simulink model "SIMQGC"  (R2017a)
settings: Solver=VariableStepAuto  StartTime=0.0  StopTime=1000  RelTol=1e-3
model workspace: external: MAT-File (data not in the file)
values from neighbouring files (symbols this model uses):
  aDe =     [MY3.mat]
  aDyn =     [MY3.mat]
  aLat =     [MY3.mat]
  aLon =     [MY3.mat]
  H = HGround + geo.Zgear + GearData.R - MCdata.mass*9.8/4/GearData.Sp    [my3_acdata.m]
  HGround = 500    [my3_acdata.m]
  phi_max = 20    [my3_acdata.m]
  phi_min = -20    [my3_acdata.m]
  psi_max = 30    [my3_acdata.m]
  psi_min = -30    [my3_acdata.m]
  theta_max = 20    [my3_acdata.m]
  theta_min = -20    [my3_acdata.m]
  Xmax = 0.01    [my3_acdata.m]
  Xmin = 0    [my3_acdata.m]
  Ymax = 0.01    [my3_acdata.m]
  Ymin = 0    [my3_acdata.m]
  Zmax = 0.01    [my3_acdata.m]
  Zmin = 0    [my3_acdata.m]
undefined symbols (not defined in the file or in its folder): Earth, geo, ini, magnitude, Motor, Newton, Prop, Raphson, Standard_Devices, UDP_Protocol, WGS84
undefined symbols (not defined in the file): GearData, LProp, RProp
libraries: simulink_extras x12, dspnetwork x8, aerolibobsolete x6, sharedutil x6, simulink x4, aerolibfltsims x3, aerolibasang x2, aerolibatmos2 x1, aerolibbdyn x1, aerolibtransform2 x1, aerolibanimutils x1, sldrtlib x1
(part 3 of 3)

== system SIMQGC/AircraftModel_MY3/Fixwing_Airframe/GroundForces/RF_Gear/detect ground contact ==
  note: height of gear lowest point
  ze : Inport
  DCM : Inport  Port=2
  Xgb : Inport  Port=3
  Hrw : Inport  Port=4
  Gain2 : Gain  Gain=-1
  Rotate pos to body axes : Product  Multiplication=Matrix(*)  SaturateOnIntegerOverflow=on  InputSameDT=on  OutDataTypeStr=Inherit: Same as first input
  Sum2 : Sum  Inputs=|++
  Sum4 : Sum  Inputs=++|
  Transpose : Math  Operator=transpose  SaturateOnIntegerOverflow=on
  Zg : Selector  InputPortWidth=3  IndexOptions=Index vector (dialog)  Indices=3  OutputSizes=1
  detect_WOW : RelationalOperator  Operator=<=  OutDataTypeStr=boolean  RndMeth=Nearest
  radius of wheel : Constant  Value=Rw  VectorParams1D=off
  WOW : Outport
  wires:
  radius of wheel/1 -> Sum2/2
  Transpose/1 -> Rotate pos to body axes/1
  Zg/1 -> Sum4/2
  Gain2/1 -> detect_WOW/1
  Sum2/1 -> Gain2/1
  Sum4/1 -> Sum2/1
  Rotate pos to body axes/1 -> Zg/1
  DCM/1 -> Transpose/1
  Xgb/1 -> Rotate pos to body axes/2
  Hrw/1 -> detect_WOW/2
  ze/1 -> Sum4/1
  detect_WOW/1 -> WOW/1

== system SIMQGC/AircraftModel_MY3/Fixwing_Airframe/PlantBus/nb & gb /cal gb ==
  DCM : Inport
  g : Inport  Port=2
  Constant2 : Constant  Value=0
  Mux : Mux  Inputs=3
  To Body Axes : Product  Multiplication=Matrix(*)  SaturateOnIntegerOverflow=on  InputSameDT=on  OutDataTypeStr=Inherit: Same as first input
  gb : Outport
  wires:
  Mux/1 -> To Body Axes/2
  Constant2/1 -> Mux/1, Mux/2
  DCM/1 -> To Body Axes/1
  To Body Axes/1 -> gb/1
  g/1 -> Mux/3

== system SIMQGC/AircraftModel_MY3/Fixwing_Airframe/Aerodynamics/Aerodynamic Coefficients/Basic Coefficients/alat ==
  beta : Inport
  alpha : Inport  Port=2
  Mux : Mux  Inputs=6
  alat_CD : Lookup_n-D  BreakpointsForDimension1=aLat.beta  BreakpointsForDimension2=aLat.alpha  Table=aLat.dCD  InternalRulePriority=Speed  RndMeth=Simplest  InputSameDT=on
  alat_CL : Lookup_n-D  BreakpointsForDimension1=aLat.beta  BreakpointsForDimension2=aLat.alpha  Table=aLat.dCL  InternalRulePriority=Speed  RndMeth=Simplest  InputSameDT=on
  alat_CY : Lookup_n-D  BreakpointsForDimension1=aLat.beta  BreakpointsForDimension2=aLat.alpha  Table=aLat.dCY  InternalRulePriority=Speed  RndMeth=Simplest  InputSameDT=on
  alat_Cl : Lookup_n-D  BreakpointsForDimension1=aLat.beta  BreakpointsForDimension2=aLat.alpha  Table=aLat.dCl  InternalRulePriority=Speed  RndMeth=Simplest  InputSameDT=on
  alat_Cm : Lookup_n-D  BreakpointsForDimension1=aLat.beta  BreakpointsForDimension2=aLat.alpha  Table=aLat.dCm  InternalRulePriority=Speed  RndMeth=Simplest  InputSameDT=on
  alat_Cn : Lookup_n-D  BreakpointsForDimension1=aLat.beta  BreakpointsForDimension2=aLat.alpha  Table=aLat.dCn  InternalRulePriority=Speed  RndMeth=Simplest  InputSameDT=on
  alat : Outport
  wires:
  beta/1 -> alat_Cn/1, alat_Cm/1, alat_Cl/1, alat_CY/1, alat_CD/1, alat_CL/1
  alpha/1 -> alat_Cn/2, alat_Cm/2, alat_Cl/2, alat_CY/2, alat_CD/2, alat_CL/2
  alat_Cm/1 -> Mux/5
  alat_CD/1 -> Mux/2
  alat_CL/1 -> Mux/1
  Mux/1 -> alat/1
  alat_CY/1 -> Mux/3
  alat_Cl/1 -> Mux/4
  alat_Cn/1 -> Mux/6

== system SIMQGC/AircraftModel_MY3/Fixwing_Airframe/Aerodynamics/Aerodynamic Coefficients/Basic Coefficients/alon ==
  alpha : Inport
  Mach : Inport  Port=2
  Constant : Constant  Value=0
  Constant1 : Constant  Value=0
  Constant2 : Constant  Value=0
  Mux : Mux  Inputs=6
  alon_CD : Lookup_n-D  BreakpointsForDimension1=aLon.alpha  BreakpointsForDimension2=aLon.mach  Table=aLon.CD  InternalRulePriority=Speed  RndMeth=Simplest  InputSameDT=on
  alon_CL : Lookup_n-D  BreakpointsForDimension1=aLon.alpha  BreakpointsForDimension2=aLon.mach  Table=aLon.CL  InternalRulePriority=Speed  RndMeth=Simplest  InputSameDT=on
  alon_Cm : Lookup_n-D  BreakpointsForDimension1=aLon.alpha  BreakpointsForDimension2=aLon.mach  Table=aLon.Cm  InternalRulePriority=Speed  RndMeth=Simplest  InputSameDT=on
  alon : Outport
  wires:
  Mux/1 -> alon/1
  alon_CL/1 -> Mux/1
  alon_CD/1 -> Mux/2
  alon_Cm/1 -> Mux/5
  Mach/1 -> alon_CL/2, alon_Cm/2, alon_CD/2
  alpha/1 -> alon_CL/1, alon_Cm/1, alon_CD/1
  Constant/1 -> Mux/3
  Constant1/1 -> Mux/4
  Constant2/1 -> Mux/6

== system SIMQGC/AircraftModel_MY3/Fixwing_Airframe/Aerodynamics/Aerodynamic Coefficients/Body Rate Damping/adyn ==
  alpha : Inport
  adyn_p : Subsystem
  adyn_q : Subsystem
  adyn_r : Subsystem
  pout : Outport
  qout : Outport  Port=2
  rout : Outport  Port=3
  wires:
  alpha/1 -> adyn_r/1(alpha), adyn_q/1(alpha), adyn_p/1(alpha)
  adyn_p/1(p) -> pout/1
  adyn_q/1(q) -> qout/1
  adyn_r/1(r) -> rout/1

== system SIMQGC/AircraftModel_MY3/Fixwing_Airframe/Aerodynamics/Aerodynamic Coefficients/actuator/ade ==
  alpha : Inport
  de : Inport  Port=2
  CD : Lookup_n-D  BreakpointsForDimension1=aDe.de  BreakpointsForDimension2=aDe.alpha  Table=aDe.dCD  InternalRulePriority=Speed  RndMeth=Simplest  InputSameDT=on
  CL : Lookup_n-D  BreakpointsForDimension1=aDe.de  BreakpointsForDimension2=aDe.alpha  Table=aDe.dCL  InternalRulePriority=Speed  RndMeth=Simplest  InputSameDT=on
  Cm : Lookup_n-D  BreakpointsForDimension1=aDe.de  BreakpointsForDimension2=aDe.alpha  Table=aDe.dCm  InternalRulePriority=Speed  RndMeth=Simplest  InputSameDT=on
  Mux2 : Mux  Inputs=6
  cld_height : Constant  Value=0
  Coeff : Outport
  wires:
  Mux2/1 -> Coeff/1
  de/1 -> Cm/1, CD/1, CL/1
  alpha/1 -> Cm/2, CD/2, CL/2
  CL/1 -> Mux2/1
  CD/1 -> Mux2/2
  cld_height/1 -> Mux2/4, Mux2/6, Mux2/3
  Cm/1 -> Mux2/5

== system SIMQGC/AircraftModel_MY3/Fixwing_Airframe/Aerodynamics/DerivedConditions1/Incidence, Sideslip, & Airspeed/Subsystem ==
  V : Inport
  Demux1 : Demux  Outputs=3
  Terminator : Terminator
  w : Outport
  U : Outport  Port=2
  wires:
  Demux1/3 -> w/1
  Demux1/2 -> Terminator/1
  V/1 -> Demux1/1
  Demux1/1 -> U/1

== system SIMQGC/AircraftModel_MY3/Fixwing_Airframe/Aerodynamics/DerivedConditions1/Incidence, Sideslip, & Airspeed/Subsystem1 ==
  V : Inport
  Demux1 : Demux  Outputs=3
  Terminator : Terminator
  Terminator1 : Terminator
  v : Outport
  wires:
  Demux1/1 -> Terminator/1
  Demux1/3 -> Terminator1/1
  V/1 -> Demux1/1
  Demux1/2 -> v/1

== system SIMQGC/AircraftModel_MY3/Fixwing_Airframe/Aerodynamics/DerivedConditions1/Incidence, Sideslip, & Airspeed/dot ==
  Vb : Inport
  Demux1 : Demux  Outputs=3
  Product : Product  RndMeth=Zero
  Product1 : Product  RndMeth=Zero
  Product2 : Product  RndMeth=Zero
  Sum : Sum  Inputs=+++
  dot : Outport
  wires:
  Product2/1 -> Sum/3
  Demux1/3 -> Product2/2, Product2/1
  Product/1 -> Sum/1
  Product1/1 -> Sum/2
  Sum/1 -> dot/1
  Vb/1 -> Demux1/1
  Demux1/1 -> Product/2, Product/1
  Demux1/2 -> Product1/1, Product1/2

== system SIMQGC/AircraftModel_MY3/Fixwing_Airframe/Aerodynamics/DerivedConditions1/gamma chi & speed/norm ==
  x : Inport
  y : Inport  Port=2
  z : Inport  Port=3
  Product1 : Product  RndMeth=Zero
  Product2 : Product  RndMeth=Zero
  Product3 : Product  RndMeth=Zero
  Sum : Sum  Inputs=+++
  speed : Math  Operator=sqrt  SaturateOnIntegerOverflow=on
  n : Outport
  wires:
  Product3/1 -> Sum/3
  Product1/1 -> Sum/1
  Product2/1 -> Sum/2
  Sum/1 -> speed/1
  speed/1 -> n/1
  x/1 -> Product1/1, Product1/2
  y/1 -> Product2/1, Product2/2
  z/1 -> Product3/1, Product3/2

== system SIMQGC/AircraftModel_MY3/Fixwing_Airframe/GroundForces/LF_Gear/GenerateGroundFM1/Calc Gear Force and Pos ==
  Xgb : Inport
  zrw : Inport  Port=2
  zcg : Inport  Port=3
  DCM : Inport  Port=4
  WgL : Inport  Port=5
  DampingRate_N/m/sec1 : Gain  Gain=Cs
  Product : Product  Multiplication=Matrix(*)
  Selector : Selector  InputPortWidth=3  IndexOptions=Index vector (dialog)  Indices=[3]  OutputSizes=1
  Selector1 : Selector  InputPortWidth=3  IndexOptions=Index vector (dialog)  Indices=[3]  OutputSizes=1
  SpringRate_N/m1 : Gain  Gain=Ks
  Sum : Sum  Inputs=+--
  Sum4 : Sum  Inputs=|-+
  Sum5 : Sum
  Transpose1 : Math  Operator=transpose  SaturateOnIntegerOverflow=on
  radius of  wheel1 : Constant  Value=Rw  VectorParams1D=off
  reaction1 : Gain  Gain=-1
  Fz1 : Outport
  S_strut1 : Outport  Port=2  InitialOutput=0
  zgb1 : Outport  Port=3  InitialOutput=0
  wires:
  DCM/1 -> Transpose1/1
  Xgb/1 -> Selector1/1, Product/2
  Transpose1/1 -> Product/1
  Product/1 -> Selector/1
  Selector/1 -> Sum/3
  zcg/1 -> Sum/2
  zrw/1 -> Sum/1
  Sum/1 -> Sum4/1
  radius of  wheel1/1 -> Sum4/2
  SpringRate_N/m1/1 -> Sum5/1
  WgL/1 -> DampingRate_N/m/sec1/1
  DampingRate_N/m/sec1/1 -> Sum5/2
  Sum5/1 -> reaction1/1  "Fstrut"
  reaction1/1 -> Fz1/1
  Selector1/1 -> zgb1/1
  Sum4/1 -> S_strut1/1, SpringRate_N/m1/1

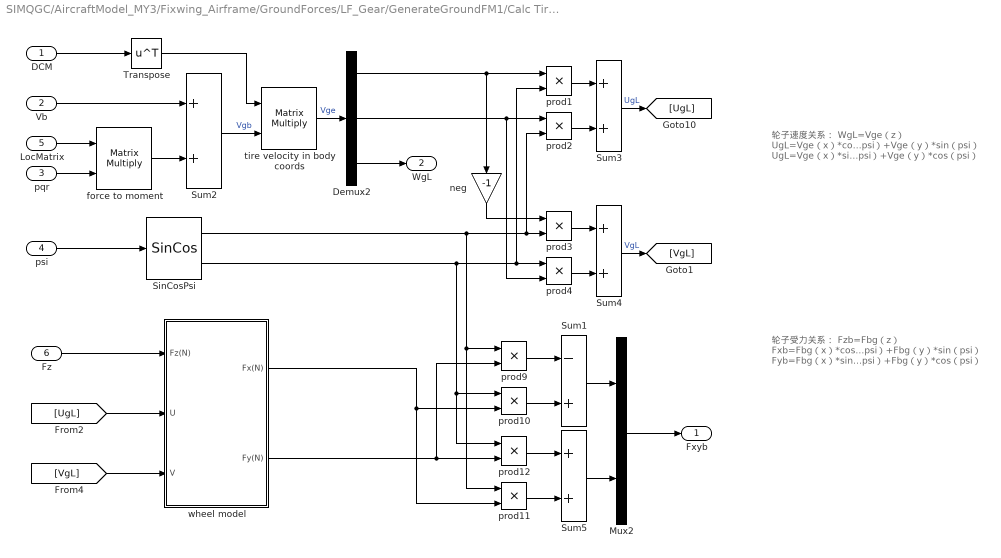
== system SIMQGC/AircraftModel_MY3/Fixwing_Airframe/GroundForces/LF_Gear/GenerateGroundFM1/Calc Tire Force ==
  note: 轮子速度关系：
      | WgL=Vge（z）
      | UgL=Vge（x）*cos（psi）+Vge（y）*sin（psi）
      | UgL=Vge（x）*sin（psi）+Vge（y）*cos（psi）
  note: 轮子受力关系：
      | Fzb=Fbg（z）
      | Fxb=Fbg（x）*cos（psi）+Fbg（y）*sin（psi）
      | Fyb=Fbg（x）*sin（psi）+Fbg（y）*cos（psi）
  DCM : Inport
  Vb : Inport  Port=2
  pqr : Inport  Port=3
  psi : Inport  Port=4
  LocMatrix : Inport  Port=5
  Fz : Inport  Port=6
  Demux2 : Demux  Outputs=3
  Mux2 : Mux  Inputs=2
  SinCosPsi : aerolibobsolete/SinCos
      settings: SourceProductName=Aerospace Blockset  SourceProductBaseCode=AE
  Sum1 : Sum  Inputs=-+
  Sum2 : Sum  Inputs=2
  Sum3 : Sum  Inputs=2
  Sum4 : Sum  Inputs=2
  Sum5 : Sum
  Transpose : Math  Operator=transpose  SaturateOnIntegerOverflow=on
  force to moment : Product  Multiplication=Matrix(*)  SaturateOnIntegerOverflow=on  InputSameDT=on  OutDataTypeStr=Inherit: Same as first input
  neg : Gain  Gain=-1
  prod{1..4,9..12} (8 alike) : Product  RndMeth=Zero
  tire velocity in body coords : Product  Multiplication=Matrix(*)  SaturateOnIntegerOverflow=on  InputSameDT=on  OutDataTypeStr=Inherit: Same as first input
  wheel model : Subsystem
  Fxyb : Outport  InitialOutput=0
  WgL : Outport  Port=2  InitialOutput=0
  wires:
  psi/1 -> SinCosPsi/1
  Sum4/1 -> [VgL]  "VgL"
  [VgL] -> wheel model/3(V)
  [UgL] -> wheel model/2(U)
  Mux2/1 -> Fxyb/1
  Sum5/1 -> Mux2/2
  Sum1/1 -> Mux2/1
  prod11/1 -> Sum5/2
  prod12/1 -> Sum5/1
  prod10/1 -> Sum1/2
  prod9/1 -> Sum1/1
  force to moment/1 -> Sum2/2
  Sum2/1 -> tire velocity in body coords/2  "Vgb"
  tire velocity in body coords/1 -> Demux2/1  "Vge"
  Demux2/1 -> neg/1, prod1/1
  Demux2/2 -> prod2/1, prod4/2
  prod1/1 -> Sum3/1
  prod2/1 -> Sum3/2
  prod3/1 -> Sum4/1
  prod4/1 -> Sum4/2
  Sum3/1 -> [UgL]  "UgL"
  neg/1 -> prod3/1
  SinCosPsi/1 -> prod11/1, prod9/1, prod2/2, prod3/2
  SinCosPsi/2 -> prod12/1, prod10/1, prod1/2, prod4/1
  Vb/1 -> Sum2/1
  LocMatrix/1 -> force to moment/1
  pqr/1 -> force to moment/2
  DCM/1 -> Transpose/1
  Transpose/1 -> tire velocity in body coords/1
  wheel model/1(Fx(N)) -> prod11/2, prod10/2
  wheel model/2(Fy(N)) -> prod9/2, prod12/2
  Fz/1 -> wheel model/1(Fz(N))
  Demux2/3 -> WgL/1

== system SIMQGC/AircraftModel_MY3/Fixwing_Airframe/GroundForces/LF_Gear/GenerateGroundFM1/LocMatrix ==
  xgb : Inport
  ygb : Inport  Port=2
  zgb : Inport  Port=3
  Create 3x3 Matrix : sharedutil/Create 3x3 Matrix
  Sum : Sum  Inputs=++|
  inv1 : Gain  Gain=-1
  inv2 : Gain  Gain=-1
  inv4 : Gain  Gain=-1
  zero1 : Constant  Value=0  SampleTime=0
  zero2 : Constant  Value=0  SampleTime=0
  zero3 : Constant  Value=0  SampleTime=0
  zero4 : Constant  Value=Rw  SampleTime=0
  A : Outport
  wires:
  xgb/1 -> Create 3x3 Matrix/6, inv2/1
  ygb/1 -> inv1/1, Create 3x3 Matrix/7
  Create 3x3 Matrix/1 -> A/1
  zero1/1 -> Create 3x3 Matrix/1
  zero2/1 -> Create 3x3 Matrix/5
  zero3/1 -> Create 3x3 Matrix/9
  inv1/1 -> Create 3x3 Matrix/3
  inv4/1 -> Create 3x3 Matrix/4
  inv2/1 -> Create 3x3 Matrix/8
  zgb/1 -> Sum/2
  zero4/1 -> Sum/1
  Sum/1 -> inv4/1, Create 3x3 Matrix/2

== system SIMQGC/AircraftModel_MY3/Fixwing_Airframe/GroundForces/LM_Gear/GenerateGroundFM1/Calc Gear Force and Pos ==
  Xgb : Inport
  zrg : Inport  Port=2
  zcg : Inport  Port=3
  DCM : Inport  Port=4
  WgL : Inport  Port=5
  DampingRate_N/m/sec1 : Gain  Gain=Cs
  Product : Product  Multiplication=Matrix(*)
  Selector : Selector  InputPortWidth=3  IndexOptions=Index vector (dialog)  Indices=[3]  OutputSizes=1
  Selector1 : Selector  InputPortWidth=3  IndexOptions=Index vector (dialog)  Indices=[3]  OutputSizes=1
  SpringRate_N/m1 : Gain  Gain=Ks
  Sum : Sum  Inputs=+--
  Sum4 : Sum  Inputs=|-+
  Sum5 : Sum
  Transpose1 : Math  Operator=transpose  SaturateOnIntegerOverflow=on
  radius of  wheel1 : Constant  Value=Rw  VectorParams1D=off
  reaction1 : Gain  Gain=-1
  Fz1 : Outport
  S_strut1 : Outport  Port=2  InitialOutput=0
  zgb1 : Outport  Port=3  InitialOutput=0
  wires:
  DCM/1 -> Transpose1/1
  Xgb/1 -> Selector1/1, Product/2
  Transpose1/1 -> Product/1
  Product/1 -> Selector/1
  Selector/1 -> Sum/3
  zcg/1 -> Sum/2
  zrg/1 -> Sum/1
  Sum/1 -> Sum4/1
  radius of  wheel1/1 -> Sum4/2
  SpringRate_N/m1/1 -> Sum5/1
  WgL/1 -> DampingRate_N/m/sec1/1
  DampingRate_N/m/sec1/1 -> Sum5/2
  Sum5/1 -> reaction1/1  "Fstrut"
  reaction1/1 -> Fz1/1
  Selector1/1 -> zgb1/1
  Sum4/1 -> S_strut1/1, SpringRate_N/m1/1

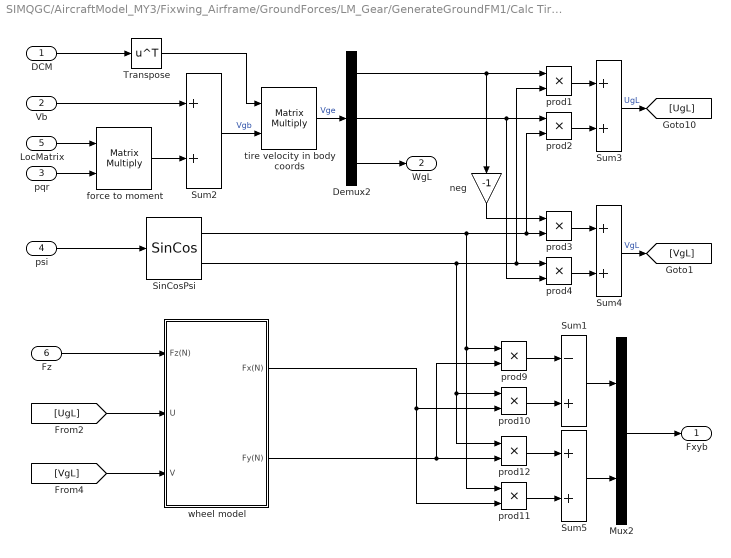
== system SIMQGC/AircraftModel_MY3/Fixwing_Airframe/GroundForces/LM_Gear/GenerateGroundFM1/Calc Tire Force ==
  DCM : Inport
  Vb : Inport  Port=2
  pqr : Inport  Port=3
  psi : Inport  Port=4
  LocMatrix : Inport  Port=5
  Fz : Inport  Port=6
  Demux2 : Demux  Outputs=3
  Mux2 : Mux  Inputs=2
  SinCosPsi : aerolibobsolete/SinCos
      settings: SourceProductName=Aerospace Blockset  SourceProductBaseCode=AE
  Sum1 : Sum  Inputs=-+
  Sum2 : Sum  Inputs=2
  Sum3 : Sum  Inputs=2
  Sum4 : Sum  Inputs=2
  Sum5 : Sum
  Transpose : Math  Operator=transpose  SaturateOnIntegerOverflow=on
  force to moment : Product  Multiplication=Matrix(*)  SaturateOnIntegerOverflow=on  InputSameDT=on  OutDataTypeStr=Inherit: Same as first input
  neg : Gain  Gain=-1
  prod{1..4,9..12} (8 alike) : Product  RndMeth=Zero
  tire velocity in body coords : Product  Multiplication=Matrix(*)  SaturateOnIntegerOverflow=on  InputSameDT=on  OutDataTypeStr=Inherit: Same as first input
  wheel model : Subsystem
  Fxyb : Outport  InitialOutput=0
  WgL : Outport  Port=2  InitialOutput=0
  wires:
  psi/1 -> SinCosPsi/1
  Sum4/1 -> [VgL]  "VgL"
  [VgL] -> wheel model/3(V)
  [UgL] -> wheel model/2(U)
  Mux2/1 -> Fxyb/1
  Sum5/1 -> Mux2/2
  Sum1/1 -> Mux2/1
  prod11/1 -> Sum5/2
  prod12/1 -> Sum5/1
  prod10/1 -> Sum1/2
  prod9/1 -> Sum1/1
  force to moment/1 -> Sum2/2
  Sum2/1 -> tire velocity in body coords/2  "Vgb"
  tire velocity in body coords/1 -> Demux2/1  "Vge"
  Demux2/1 -> neg/1, prod1/1
  Demux2/2 -> prod2/1, prod4/2
  prod1/1 -> Sum3/1
  prod2/1 -> Sum3/2
  prod3/1 -> Sum4/1
  prod4/1 -> Sum4/2
  Sum3/1 -> [UgL]  "UgL"
  neg/1 -> prod3/1
  SinCosPsi/1 -> prod11/1, prod9/1, prod2/2, prod3/2
  SinCosPsi/2 -> prod12/1, prod10/1, prod1/2, prod4/1
  Vb/1 -> Sum2/1
  LocMatrix/1 -> force to moment/1
  pqr/1 -> force to moment/2
  DCM/1 -> Transpose/1
  Transpose/1 -> tire velocity in body coords/1
  wheel model/1(Fx(N)) -> prod11/2, prod10/2
  wheel model/2(Fy(N)) -> prod9/2, prod12/2
  Fz/1 -> wheel model/1(Fz(N))
  Demux2/3 -> WgL/1

== system SIMQGC/AircraftModel_MY3/Fixwing_Airframe/GroundForces/LM_Gear/GenerateGroundFM1/LocMatrix ==
  xgb : Inport
  ygb : Inport  Port=2
  zgb : Inport  Port=3
  Create 3x3 Matrix : sharedutil/Create 3x3 Matrix
  Sum : Sum  Inputs=++|
  inv1 : Gain  Gain=-1
  inv2 : Gain  Gain=-1
  inv4 : Gain  Gain=-1
  zero1 : Constant  Value=0  SampleTime=0
  zero2 : Constant  Value=0  SampleTime=0
  zero3 : Constant  Value=0  SampleTime=0
  zero4 : Constant  Value=Rw  SampleTime=0
  A : Outport
  wires:
  xgb/1 -> Create 3x3 Matrix/6, inv2/1
  ygb/1 -> inv1/1, Create 3x3 Matrix/7
  Create 3x3 Matrix/1 -> A/1
  zero1/1 -> Create 3x3 Matrix/1
  zero2/1 -> Create 3x3 Matrix/5
  zero3/1 -> Create 3x3 Matrix/9
  inv1/1 -> Create 3x3 Matrix/3
  inv4/1 -> Create 3x3 Matrix/4
  inv2/1 -> Create 3x3 Matrix/8
  zgb/1 -> Sum/2
  zero4/1 -> Sum/1
  Sum/1 -> inv4/1, Create 3x3 Matrix/2

== system SIMQGC/AircraftModel_MY3/Fixwing_Airframe/GroundForces/LN_Gear/GenerateGroundFM1/Calc Gear Force and Pos ==
  Xgb : Inport
  zrg : Inport  Port=2
  zcg : Inport  Port=3
  DCM : Inport  Port=4
  WgL : Inport  Port=5
  DampingRate_N/m/sec1 : Gain  Gain=Cs
  Product : Product  Multiplication=Matrix(*)
  Selector : Selector  InputPortWidth=3  IndexOptions=Index vector (dialog)  Indices=[3]  OutputSizes=1
  Selector1 : Selector  InputPortWidth=3  IndexOptions=Index vector (dialog)  Indices=[3]  OutputSizes=1
  SpringRate_N/m1 : Gain  Gain=Ks
  Sum : Sum  Inputs=+--
  Sum4 : Sum  Inputs=|-+
  Sum5 : Sum
  Transpose1 : Math  Operator=transpose  SaturateOnIntegerOverflow=on
  radius of  wheel1 : Constant  Value=Rw  VectorParams1D=off
  reaction1 : Gain  Gain=-1
  Fz1 : Outport
  S_strut1 : Outport  Port=2  InitialOutput=0
  zgb1 : Outport  Port=3  InitialOutput=0
  wires:
  DCM/1 -> Transpose1/1
  Xgb/1 -> Selector1/1, Product/2
  Transpose1/1 -> Product/1
  Product/1 -> Selector/1
  Selector/1 -> Sum/3
  zcg/1 -> Sum/2
  zrg/1 -> Sum/1
  Sum/1 -> Sum4/1
  radius of  wheel1/1 -> Sum4/2
  SpringRate_N/m1/1 -> Sum5/1
  WgL/1 -> DampingRate_N/m/sec1/1
  DampingRate_N/m/sec1/1 -> Sum5/2
  Sum5/1 -> reaction1/1  "Fstrut"
  reaction1/1 -> Fz1/1
  Selector1/1 -> zgb1/1
  Sum4/1 -> S_strut1/1, SpringRate_N/m1/1

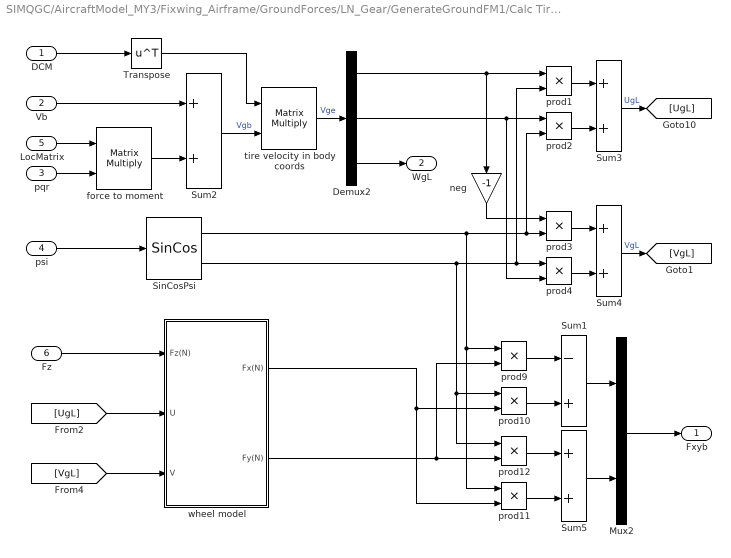
== system SIMQGC/AircraftModel_MY3/Fixwing_Airframe/GroundForces/LN_Gear/GenerateGroundFM1/Calc Tire Force ==
  DCM : Inport
  Vb : Inport  Port=2
  pqr : Inport  Port=3
  psi : Inport  Port=4
  LocMatrix : Inport  Port=5
  Fz : Inport  Port=6
  Demux2 : Demux  Outputs=3
  Mux2 : Mux  Inputs=2
  SinCosPsi : aerolibobsolete/SinCos
      settings: SourceProductName=Aerospace Blockset  SourceProductBaseCode=AE
  Sum1 : Sum  Inputs=-+
  Sum2 : Sum  Inputs=2
  Sum3 : Sum  Inputs=2
  Sum4 : Sum  Inputs=2
  Sum5 : Sum
  Transpose : Math  Operator=transpose  SaturateOnIntegerOverflow=on
  force to moment : Product  Multiplication=Matrix(*)  SaturateOnIntegerOverflow=on  InputSameDT=on  OutDataTypeStr=Inherit: Same as first input
  neg : Gain  Gain=-1
  prod{1..4,9..12} (8 alike) : Product  RndMeth=Zero
  tire velocity in body coords : Product  Multiplication=Matrix(*)  SaturateOnIntegerOverflow=on  InputSameDT=on  OutDataTypeStr=Inherit: Same as first input
  wheel model : Subsystem
  Fxyb : Outport  InitialOutput=0
  WgL : Outport  Port=2  InitialOutput=0
  wires:
  psi/1 -> SinCosPsi/1
  Sum4/1 -> [VgL]  "VgL"
  [VgL] -> wheel model/3(V)
  [UgL] -> wheel model/2(U)
  Mux2/1 -> Fxyb/1
  Sum5/1 -> Mux2/2
  Sum1/1 -> Mux2/1
  prod11/1 -> Sum5/2
  prod12/1 -> Sum5/1
  prod10/1 -> Sum1/2
  prod9/1 -> Sum1/1
  force to moment/1 -> Sum2/2
  Sum2/1 -> tire velocity in body coords/2  "Vgb"
  tire velocity in body coords/1 -> Demux2/1  "Vge"
  Demux2/1 -> neg/1, prod1/1
  Demux2/2 -> prod2/1, prod4/2
  prod1/1 -> Sum3/1
  prod2/1 -> Sum3/2
  prod3/1 -> Sum4/1
  prod4/1 -> Sum4/2
  Sum3/1 -> [UgL]  "UgL"
  neg/1 -> prod3/1
  SinCosPsi/1 -> prod11/1, prod9/1, prod2/2, prod3/2
  SinCosPsi/2 -> prod12/1, prod10/1, prod1/2, prod4/1
  Vb/1 -> Sum2/1
  LocMatrix/1 -> force to moment/1
  pqr/1 -> force to moment/2
  DCM/1 -> Transpose/1
  Transpose/1 -> tire velocity in body coords/1
  wheel model/1(Fx(N)) -> prod11/2, prod10/2
  wheel model/2(Fy(N)) -> prod9/2, prod12/2
  Fz/1 -> wheel model/1(Fz(N))
  Demux2/3 -> WgL/1

== system SIMQGC/AircraftModel_MY3/Fixwing_Airframe/GroundForces/LN_Gear/GenerateGroundFM1/LocMatrix ==
  xgb : Inport
  ygb : Inport  Port=2
  zgb : Inport  Port=3
  Create 3x3 Matrix : sharedutil/Create 3x3 Matrix
  Sum : Sum  Inputs=++|
  inv1 : Gain  Gain=-1
  inv2 : Gain  Gain=-1
  inv4 : Gain  Gain=-1
  zero1 : Constant  Value=0  SampleTime=0
  zero2 : Constant  Value=0  SampleTime=0
  zero3 : Constant  Value=0  SampleTime=0
  zero4 : Constant  Value=Rw  SampleTime=0
  A : Outport
  wires:
  xgb/1 -> Create 3x3 Matrix/6, inv2/1
  ygb/1 -> inv1/1, Create 3x3 Matrix/7
  Create 3x3 Matrix/1 -> A/1
  zero1/1 -> Create 3x3 Matrix/1
  zero2/1 -> Create 3x3 Matrix/5
  zero3/1 -> Create 3x3 Matrix/9
  inv1/1 -> Create 3x3 Matrix/3
  inv4/1 -> Create 3x3 Matrix/4
  inv2/1 -> Create 3x3 Matrix/8
  zgb/1 -> Sum/2
  zero4/1 -> Sum/1
  Sum/1 -> inv4/1, Create 3x3 Matrix/2

== system SIMQGC/AircraftModel_MY3/Fixwing_Airframe/GroundForces/RF_Gear/GenerateGroundFM1/Calc Gear Force and Pos ==
  Xgb : Inport
  zrg : Inport  Port=2
  zcg : Inport  Port=3
  DCM : Inport  Port=4
  WgL : Inport  Port=5
  DampingRate_N/m/sec1 : Gain  Gain=Cs
  Product : Product  Multiplication=Matrix(*)
  Selector : Selector  InputPortWidth=3  IndexOptions=Index vector (dialog)  Indices=[3]  OutputSizes=1
  Selector1 : Selector  InputPortWidth=3  IndexOptions=Index vector (dialog)  Indices=[3]  OutputSizes=1
  SpringRate_N/m1 : Gain  Gain=Ks
  Sum : Sum  Inputs=+--
  Sum4 : Sum  Inputs=|-+
  Sum5 : Sum
  Transpose1 : Math  Operator=transpose  SaturateOnIntegerOverflow=on
  radius of  wheel1 : Constant  Value=Rw  VectorParams1D=off
  reaction1 : Gain  Gain=-1
  Fz1 : Outport
  S_strut1 : Outport  Port=2  InitialOutput=0
  zgb1 : Outport  Port=3  InitialOutput=0
  wires:
  DCM/1 -> Transpose1/1
  Xgb/1 -> Selector1/1, Product/2
  Transpose1/1 -> Product/1
  Product/1 -> Selector/1
  Selector/1 -> Sum/3
  zcg/1 -> Sum/2
  zrg/1 -> Sum/1
  Sum/1 -> Sum4/1
  radius of  wheel1/1 -> Sum4/2
  SpringRate_N/m1/1 -> Sum5/1
  WgL/1 -> DampingRate_N/m/sec1/1
  DampingRate_N/m/sec1/1 -> Sum5/2
  Sum5/1 -> reaction1/1  "Fstrut"
  reaction1/1 -> Fz1/1
  Selector1/1 -> zgb1/1
  Sum4/1 -> S_strut1/1, SpringRate_N/m1/1

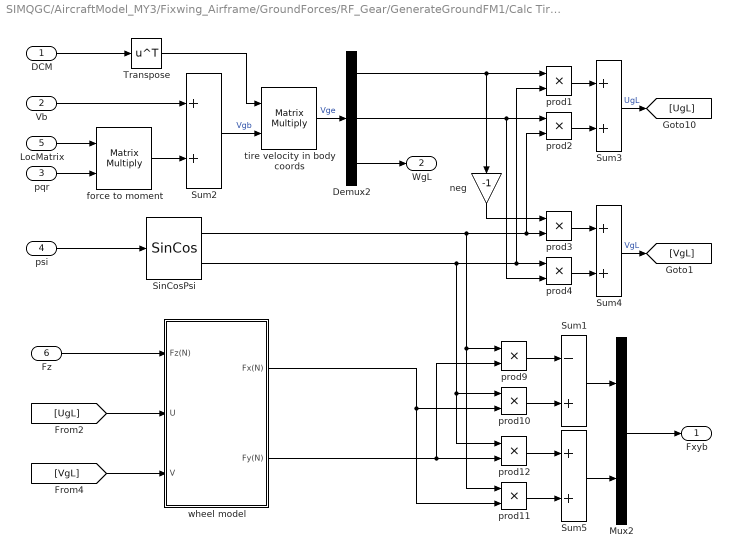
== system SIMQGC/AircraftModel_MY3/Fixwing_Airframe/GroundForces/RF_Gear/GenerateGroundFM1/Calc Tire Force ==
  DCM : Inport
  Vb : Inport  Port=2
  pqr : Inport  Port=3
  psi : Inport  Port=4
  LocMatrix : Inport  Port=5
  Fz : Inport  Port=6
  Demux2 : Demux  Outputs=3
  Mux2 : Mux  Inputs=2
  SinCosPsi : aerolibobsolete/SinCos
      settings: SourceProductName=Aerospace Blockset  SourceProductBaseCode=AE
  Sum1 : Sum  Inputs=-+
  Sum2 : Sum  Inputs=2
  Sum3 : Sum  Inputs=2
  Sum4 : Sum  Inputs=2
  Sum5 : Sum
  Transpose : Math  Operator=transpose  SaturateOnIntegerOverflow=on
  force to moment : Product  Multiplication=Matrix(*)  SaturateOnIntegerOverflow=on  InputSameDT=on  OutDataTypeStr=Inherit: Same as first input
  neg : Gain  Gain=-1
  prod{1..4,9..12} (8 alike) : Product  RndMeth=Zero
  tire velocity in body coords : Product  Multiplication=Matrix(*)  SaturateOnIntegerOverflow=on  InputSameDT=on  OutDataTypeStr=Inherit: Same as first input
  wheel model : Subsystem
  Fxyb : Outport  InitialOutput=0
  WgL : Outport  Port=2  InitialOutput=0
  wires:
  psi/1 -> SinCosPsi/1
  Sum4/1 -> [VgL]  "VgL"
  [VgL] -> wheel model/3(V)
  [UgL] -> wheel model/2(U)
  Mux2/1 -> Fxyb/1
  Sum5/1 -> Mux2/2
  Sum1/1 -> Mux2/1
  prod11/1 -> Sum5/2
  prod12/1 -> Sum5/1
  prod10/1 -> Sum1/2
  prod9/1 -> Sum1/1
  force to moment/1 -> Sum2/2
  Sum2/1 -> tire velocity in body coords/2  "Vgb"
  tire velocity in body coords/1 -> Demux2/1  "Vge"
  Demux2/1 -> neg/1, prod1/1
  Demux2/2 -> prod2/1, prod4/2
  prod1/1 -> Sum3/1
  prod2/1 -> Sum3/2
  prod3/1 -> Sum4/1
  prod4/1 -> Sum4/2
  Sum3/1 -> [UgL]  "UgL"
  neg/1 -> prod3/1
  SinCosPsi/1 -> prod11/1, prod9/1, prod2/2, prod3/2
  SinCosPsi/2 -> prod12/1, prod10/1, prod1/2, prod4/1
  Vb/1 -> Sum2/1
  LocMatrix/1 -> force to moment/1
  pqr/1 -> force to moment/2
  DCM/1 -> Transpose/1
  Transpose/1 -> tire velocity in body coords/1
  wheel model/1(Fx(N)) -> prod11/2, prod10/2
  wheel model/2(Fy(N)) -> prod9/2, prod12/2
  Fz/1 -> wheel model/1(Fz(N))
  Demux2/3 -> WgL/1

== system SIMQGC/AircraftModel_MY3/Fixwing_Airframe/GroundForces/RF_Gear/GenerateGroundFM1/LocMatrix ==
  xgb : Inport
  ygb : Inport  Port=2
  zgb : Inport  Port=3
  Create 3x3 Matrix : sharedutil/Create 3x3 Matrix
  Sum : Sum  Inputs=++|
  inv1 : Gain  Gain=-1
  inv2 : Gain  Gain=-1
  inv4 : Gain  Gain=-1
  zero1 : Constant  Value=0  SampleTime=0
  zero2 : Constant  Value=0  SampleTime=0
  zero3 : Constant  Value=0  SampleTime=0
  zero4 : Constant  Value=Rw  SampleTime=0
  A : Outport
  wires:
  xgb/1 -> Create 3x3 Matrix/6, inv2/1
  ygb/1 -> inv1/1, Create 3x3 Matrix/7
  Create 3x3 Matrix/1 -> A/1
  zero1/1 -> Create 3x3 Matrix/1
  zero2/1 -> Create 3x3 Matrix/5
  zero3/1 -> Create 3x3 Matrix/9
  inv1/1 -> Create 3x3 Matrix/3
  inv4/1 -> Create 3x3 Matrix/4
  inv2/1 -> Create 3x3 Matrix/8
  zgb/1 -> Sum/2
  zero4/1 -> Sum/1
  Sum/1 -> inv4/1, Create 3x3 Matrix/2

== system SIMQGC/AircraftModel_MY3/Fixwing_Airframe/Aerodynamics/Aerodynamic Coefficients/Body Rate Damping/adyn/adyn_p ==
  alpha : Inport
  Constant : Constant  Value=0
  Mux : Mux  Inputs=6
  Yp : Lookup_n-D  NumberOfTableDimensions=1  BreakpointsForDimension1=aDyn.alpha  Table=aDyn.CYp  InternalRulePriority=Speed  RndMeth=Simplest  InputSameDT=on
  lp : Lookup_n-D  NumberOfTableDimensions=1  BreakpointsForDimension1=aDyn.alpha  Table=aDyn.Clp  InternalRulePriority=Speed  RndMeth=Simplest  InputSameDT=on
  np : Lookup_n-D  NumberOfTableDimensions=1  BreakpointsForDimension1=aDyn.alpha  Table=aDyn.Cnp  InternalRulePriority=Speed  RndMeth=Simplest  InputSameDT=on
  p : Outport
  wires:
  lp/1 -> Mux/4
  Yp/1 -> Mux/3
  np/1 -> Mux/6
  alpha/1 -> np/1, lp/1, Yp/1
  Constant/1 -> Mux/1, Mux/2, Mux/5
  Mux/1 -> p/1

== system SIMQGC/AircraftModel_MY3/Fixwing_Airframe/Aerodynamics/Aerodynamic Coefficients/Body Rate Damping/adyn/adyn_q ==
  alpha : Inport
  Constant : Constant  Value=0
  Dq : Lookup_n-D  NumberOfTableDimensions=1  BreakpointsForDimension1=aDyn.alpha  Table=aDyn.CDq  InternalRulePriority=Speed  RndMeth=Simplest  InputSameDT=on
  Lq : Lookup_n-D  NumberOfTableDimensions=1  BreakpointsForDimension1=aDyn.alpha  Table=aDyn.CLq  InternalRulePriority=Speed  RndMeth=Simplest  InputSameDT=on
  Mq : Lookup_n-D  NumberOfTableDimensions=1  BreakpointsForDimension1=aDyn.alpha  Table=aDyn.Cmq  InternalRulePriority=Speed  RndMeth=Simplest  InputSameDT=on
  Mux : Mux  Inputs=6
  q : Outport
  wires:
  Mux/1 -> q/1
  alpha/1 -> Mq/1, Dq/1, Lq/1
  Lq/1 -> Mux/1
  Dq/1 -> Mux/2
  Mq/1 -> Mux/5
  Constant/1 -> Mux/6, Mux/4, Mux/3

== system SIMQGC/AircraftModel_MY3/Fixwing_Airframe/Aerodynamics/Aerodynamic Coefficients/Body Rate Damping/adyn/adyn_r ==
  alpha : Inport
  Constant : Constant  Value=0
  Mux : Mux  Inputs=6
  Yr : Lookup_n-D  NumberOfTableDimensions=1  BreakpointsForDimension1=aDyn.alpha  Table=aDyn.CYr  InternalRulePriority=Speed  RndMeth=Simplest  InputSameDT=on
  lr : Lookup_n-D  NumberOfTableDimensions=1  BreakpointsForDimension1=aDyn.alpha  Table=aDyn.Clr  InternalRulePriority=Speed  RndMeth=Simplest  InputSameDT=on
  nr : Lookup_n-D  NumberOfTableDimensions=1  BreakpointsForDimension1=aDyn.alpha  Table=aDyn.Cnr  InternalRulePriority=Speed  RndMeth=Simplest  InputSameDT=on
  r : Outport
  wires:
  Mux/1 -> r/1
  Constant/1 -> Mux/5, Mux/2, Mux/1
  alpha/1 -> Yr/1, nr/1, lr/1
  nr/1 -> Mux/6
  Yr/1 -> Mux/3
  lr/1 -> Mux/4

== system SIMQGC/AircraftModel_MY3/Fixwing_Airframe/GroundForces/LF_Gear/GenerateGroundFM1/Calc Tire Force/wheel model ==
  note: simple wheel model
      | no wheel model and brake device model
      | not consider slip ratio caused forces
  Fz(N) : Inport
  U : Inport  Port=2
  V : Inport  Port=3
  Abs : Abs  ZeroCross=off
  Abs1 : Abs
  Gain : Gain  Gain=-1
  Gain1 : Gain  Gain=-1
  Gain2 : Gain  Gain=-1
  Product1 : Product  SaturateOnIntegerOverflow=on  InputSameDT=on  OutDataTypeStr=Inherit: Same as first input
  Product2 : Product  SaturateOnIntegerOverflow=on  InputSameDT=on  OutDataTypeStr=Inherit: Same as first input
  Product3 : Product  SaturateOnIntegerOverflow=on  InputSameDT=on  OutDataTypeStr=Inherit: Same as first input
  Saturation : Saturate  UpperLimit=10  LowerLimit=-10
  Sign : Signum  ZeroCross=off
  Switch : Switch  Threshold=0.01  ZeroCross=off
  cal side slipe angle : Subsystem
  lateral force: A*beta*(1-B*beta^2) : Fcn  Expr=A*u[1]*(1-B*u[1]*u[1])
  roll friction conefficient : Constant  Value=muroll
  Fx(N) : Outport
  Fy(N) : Outport  Port=2
  wires:
  Product2/1 -> Fy(N)/1
  Switch/1 -> Fx(N)/1
  Gain1/1 -> Product2/2
  lateral force: A*beta*(1-B*beta^2)/1 -> Gain1/1
  Saturation/1 -> lateral force: A*beta*(1-B*beta^2)/1
  V/1 -> cal side slipe angle/2(v)
  Product1/1 -> Switch/1
  Abs1/1 -> Switch/2
  Gain2/1 -> Switch/3
  Gain/1 -> Product1/2
  Abs/1 -> Product2/1, Product3/2
  Sign/1 -> Gain/1
  Product3/1 -> Product1/1
  U/1 -> cal side slipe angle/1(u), Abs1/1, Gain2/1, Sign/1
  roll friction conefficient/1 -> Product3/1
  Fz(N)/1 -> Abs/1
  cal side slipe angle/1(betae) -> Saturation/1

== system SIMQGC/AircraftModel_MY3/Fixwing_Airframe/GroundForces/LM_Gear/GenerateGroundFM1/Calc Tire Force/wheel model ==
  note: simple wheel model
      | no wheel model and brake device model
      | not consider slip ratio caused forces
  Fz(N) : Inport
  U : Inport  Port=2
  V : Inport  Port=3
  Abs : Abs  ZeroCross=off
  Abs1 : Abs
  Gain : Gain  Gain=-1
  Gain1 : Gain  Gain=-1
  Gain2 : Gain  Gain=-1
  Product1 : Product  SaturateOnIntegerOverflow=on  InputSameDT=on  OutDataTypeStr=Inherit: Same as first input
  Product2 : Product  SaturateOnIntegerOverflow=on  InputSameDT=on  OutDataTypeStr=Inherit: Same as first input
  Product3 : Product  SaturateOnIntegerOverflow=on  InputSameDT=on  OutDataTypeStr=Inherit: Same as first input
  Saturation : Saturate  UpperLimit=10  LowerLimit=-10
  Sign : Signum  ZeroCross=off
  Switch : Switch  Threshold=0.01  ZeroCross=off
  cal side slipe angle : Subsystem
  lateral force: A*beta*(1-B*beta^2) : Fcn  Expr=A*u[1]*(1-B*u[1]*u[1])
  roll friction conefficient : Constant  Value=muroll
  Fx(N) : Outport
  Fy(N) : Outport  Port=2
  wires:
  Product2/1 -> Fy(N)/1
  Switch/1 -> Fx(N)/1
  Gain1/1 -> Product2/2
  lateral force: A*beta*(1-B*beta^2)/1 -> Gain1/1
  Saturation/1 -> lateral force: A*beta*(1-B*beta^2)/1
  V/1 -> cal side slipe angle/2(v)
  Product1/1 -> Switch/1
  Abs1/1 -> Switch/2
  Gain2/1 -> Switch/3
  Gain/1 -> Product1/2
  Abs/1 -> Product2/1, Product3/2
  Sign/1 -> Gain/1
  Product3/1 -> Product1/1
  U/1 -> cal side slipe angle/1(u), Abs1/1, Gain2/1, Sign/1
  roll friction conefficient/1 -> Product3/1
  Fz(N)/1 -> Abs/1
  cal side slipe angle/1(betae) -> Saturation/1

== system SIMQGC/AircraftModel_MY3/Fixwing_Airframe/GroundForces/LN_Gear/GenerateGroundFM1/Calc Tire Force/wheel model ==
  note: simple wheel model
      | no wheel model and brake device model
      | not consider slip ratio caused forces
  Fz(N) : Inport
  U : Inport  Port=2
  V : Inport  Port=3
  Abs : Abs  ZeroCross=off
  Abs1 : Abs
  Gain : Gain  Gain=-1
  Gain1 : Gain  Gain=-1
  Gain2 : Gain  Gain=-1
  Product1 : Product  SaturateOnIntegerOverflow=on  InputSameDT=on  OutDataTypeStr=Inherit: Same as first input
  Product2 : Product  SaturateOnIntegerOverflow=on  InputSameDT=on  OutDataTypeStr=Inherit: Same as first input
  Product3 : Product  SaturateOnIntegerOverflow=on  InputSameDT=on  OutDataTypeStr=Inherit: Same as first input
  Saturation : Saturate  UpperLimit=10  LowerLimit=-10
  Sign : Signum  ZeroCross=off
  Switch : Switch  Threshold=0.01  ZeroCross=off
  cal side slipe angle : Subsystem
  lateral force: A*beta*(1-B*beta^2) : Fcn  Expr=A*u[1]*(1-B*u[1]*u[1])
  roll friction conefficient : Constant  Value=muroll
  Fx(N) : Outport
  Fy(N) : Outport  Port=2
  wires:
  Product2/1 -> Fy(N)/1
  Switch/1 -> Fx(N)/1
  Gain1/1 -> Product2/2
  lateral force: A*beta*(1-B*beta^2)/1 -> Gain1/1
  Saturation/1 -> lateral force: A*beta*(1-B*beta^2)/1
  V/1 -> cal side slipe angle/2(v)
  Product1/1 -> Switch/1
  Abs1/1 -> Switch/2
  Gain2/1 -> Switch/3
  Gain/1 -> Product1/2
  Abs/1 -> Product2/1, Product3/2
  Sign/1 -> Gain/1
  Product3/1 -> Product1/1
  U/1 -> cal side slipe angle/1(u), Abs1/1, Gain2/1, Sign/1
  roll friction conefficient/1 -> Product3/1
  Fz(N)/1 -> Abs/1
  cal side slipe angle/1(betae) -> Saturation/1

== system SIMQGC/AircraftModel_MY3/Fixwing_Airframe/GroundForces/RF_Gear/GenerateGroundFM1/Calc Tire Force/wheel model ==
  note: simple wheel model
      | no wheel model and brake device model
      | not consider slip ratio caused forces
  Fz(N) : Inport
  U : Inport  Port=2
  V : Inport  Port=3
  Abs : Abs  ZeroCross=off
  Abs1 : Abs
  Gain : Gain  Gain=-1
  Gain1 : Gain  Gain=-1
  Gain2 : Gain  Gain=-1
  Product1 : Product  SaturateOnIntegerOverflow=on  InputSameDT=on  OutDataTypeStr=Inherit: Same as first input
  Product2 : Product  SaturateOnIntegerOverflow=on  InputSameDT=on  OutDataTypeStr=Inherit: Same as first input
  Product3 : Product  SaturateOnIntegerOverflow=on  InputSameDT=on  OutDataTypeStr=Inherit: Same as first input
  Saturation : Saturate  UpperLimit=10  LowerLimit=-10
  Sign : Signum  ZeroCross=off
  Switch : Switch  Threshold=0.01  ZeroCross=off
  cal side slipe angle : Subsystem
  lateral force: A*beta*(1-B*beta^2) : Fcn  Expr=A*u[1]*(1-B*u[1]*u[1])
  roll friction conefficient : Constant  Value=muroll
  Fx(N) : Outport
  Fy(N) : Outport  Port=2
  wires:
  Product2/1 -> Fy(N)/1
  Switch/1 -> Fx(N)/1
  Gain1/1 -> Product2/2
  lateral force: A*beta*(1-B*beta^2)/1 -> Gain1/1
  Saturation/1 -> lateral force: A*beta*(1-B*beta^2)/1
  V/1 -> cal side slipe angle/2(v)
  Product1/1 -> Switch/1
  Abs1/1 -> Switch/2
  Gain2/1 -> Switch/3
  Gain/1 -> Product1/2
  Abs/1 -> Product2/1, Product3/2
  Sign/1 -> Gain/1
  Product3/1 -> Product1/1
  U/1 -> cal side slipe angle/1(u), Abs1/1, Gain2/1, Sign/1
  roll friction conefficient/1 -> Product3/1
  Fz(N)/1 -> Abs/1
  cal side slipe angle/1(betae) -> Saturation/1

== system SIMQGC/AircraftModel_MY3/Fixwing_Airframe/GroundForces/LF_Gear/GenerateGroundFM1/Calc Tire Force/wheel model/cal side slipe angle ==
  note: u>0.01
  u : Inport
  v : Inport  Port=2
  Saturation : Saturate  UpperLimit=inf  LowerLimit=1
  Trigonometric Function : Trigonometry  Operator=atan2
  betae : Outport
  wires:
  u/1 -> Saturation/1
  Saturation/1 -> Trigonometric Function/2
  Trigonometric Function/1 -> betae/1
  v/1 -> Trigonometric Function/1

== system SIMQGC/AircraftModel_MY3/Fixwing_Airframe/GroundForces/LM_Gear/GenerateGroundFM1/Calc Tire Force/wheel model/cal side slipe angle ==
  note: u>0.01
  u : Inport
  v : Inport  Port=2
  Saturation : Saturate  UpperLimit=inf  LowerLimit=1
  Trigonometric Function : Trigonometry  Operator=atan2
  betae : Outport
  wires:
  u/1 -> Saturation/1
  Saturation/1 -> Trigonometric Function/2
  Trigonometric Function/1 -> betae/1
  v/1 -> Trigonometric Function/1

== system SIMQGC/AircraftModel_MY3/Fixwing_Airframe/GroundForces/LN_Gear/GenerateGroundFM1/Calc Tire Force/wheel model/cal side slipe angle ==
  note: u>0.01
  u : Inport
  v : Inport  Port=2
  Saturation : Saturate  UpperLimit=inf  LowerLimit=1
  Trigonometric Function : Trigonometry  Operator=atan2
  betae : Outport
  wires:
  u/1 -> Saturation/1
  Saturation/1 -> Trigonometric Function/2
  Trigonometric Function/1 -> betae/1
  v/1 -> Trigonometric Function/1

== system SIMQGC/AircraftModel_MY3/Fixwing_Airframe/GroundForces/RF_Gear/GenerateGroundFM1/Calc Tire Force/wheel model/cal side slipe angle ==
  note: u>0.01
  u : Inport
  v : Inport  Port=2
  Saturation : Saturate  UpperLimit=inf  LowerLimit=1
  Trigonometric Function : Trigonometry  Operator=atan2
  betae : Outport
  wires:
  u/1 -> Saturation/1
  Saturation/1 -> Trigonometric Function/2
  Trigonometric Function/1 -> betae/1
  v/1 -> Trigonometric Function/1

== matlab function SIMQGC/UDPSendToQGC/UDP_send 3 /Byte Pack ==
  data: head input; OUT output; index input; data input
function OUT = data_transfer_uint8(head,index,data)
OUT = uint8(zeros(41,1));
OUT(1 : 5) = uint8(head);
OUT(6) = uint8(index);
OUT(10:41) = typecast(single(data),'uint8');
end

== matlab function SIMQGC/UDPSendToQGC/UDP_send 4/Byte Pack ==
  data: head input; OUT output; index input; data input
function OUT = data_transfer_uint8(head,index,data)
OUT = uint8(zeros(41,1));
OUT(1 : 5) = uint8(head);
OUT(6) = uint8(index);
OUT(10:41) = typecast(single(data),'uint8');
end

== matlab function SIMQGC/UDPSendToQGC/UDP_send 6/Byte Pack ==
  data: head input; OUT output; index input; data input
function OUT = data_transfer_uint8(head,index,data)
OUT = uint8(zeros(41,1));
OUT(1 : 5) = uint8(head);
OUT(6) = uint8(index);
OUT(10:41) = typecast(single(data),'uint8');
end

== matlab function SIMQGC/UDPSendToQGC/UDP_send 16/Byte Pack ==
  data: head input; OUT output; index input; data input
function OUT = data_transfer_uint8(head,index,data)
OUT = uint8(zeros(41,1));
OUT(1 : 5) = uint8(head);
OUT(6) = uint8(index);
OUT(10:41) = typecast(single(data),'uint8');
end

== matlab function SIMQGC/UDPSendToQGC/UDP_send 17/Byte Pack ==
  data: head input; OUT output; index input; data input
function OUT = data_transfer_uint8(head,index,data)
OUT = uint8(zeros(41,1));
OUT(1 : 5) = uint8(head);
OUT(6) = uint8(index);
OUT(10:41) = typecast(single(data),'uint8');
end

== matlab function SIMQGC/UDPSendToQGC/UDP_send 20/Byte Pack ==
  data: head input; OUT output; index input; data input
function OUT = data_transfer_uint8(head,index,data)
OUT = uint8(zeros(41,1));
OUT(1 : 5) = uint8(head);
OUT(6) = uint8(index);
OUT(10:41) = typecast(single(data),'uint8');
end

== matlab function SIMQGC/UDPSendToQGC/UDP_send 21/Byte Pack ==
  data: head input; OUT output; index input; data input
function OUT = data_transfer_uint8(head,index,data)
OUT = uint8(zeros(41,1));
OUT(1 : 5) = uint8(head);
OUT(6) = uint8(index);
OUT(10:41) = typecast(single(data),'uint8');
end

== matlab function SIMQGC/Controller/MATLAB Function ==
  data: H input; phic output
function phic = fcn(H)

if H < 545
    phic = 0;
else
    phic = 10;
end

== matlab function SIMQGC/toUDP/draw pyr ==
  data: u input; y output
function y = fcn(u)
figure;
subplot(3,1,1);plot(u(1),'LineWidth',2);set(gca,'color','none');
subplot(3,1,2);plot(u(2),'LineWidth',2);set(gca,'color','none');
subplot(3,1,3);plot(u(3),'LineWidth',2);set(gca,'color','none');
y = u;

== matlab function SIMQGC/toUDP/draw xyz ==
  data: u input; y output
function y = fcn(u)
figure;
subplot(3,1,1);plot(u(1),'LineWidth',2);set(gca,'color','none');
subplot(3,1,2);plot(u(2),'LineWidth',2);set(gca,'color','none');
subplot(3,1,3);plot(u(3),'LineWidth',2);set(gca,'color','none');
y = u;

== matlab function SIMQGC/UDPReadFromQGC/Subsystem/MATLAB Function ==
  data: a input; data output; length input
function data = fcn(a, length)
% if size(a,2) == 41
%     U= a(1,1:41);
% else
%     U= uint8(zeros(1,41));
% end

if length == 41
    data = a;
else
    data= uint8(zeros(41,1));
end
% if a(1,1) == uint8(68) && a(2,1) == uint8(65)
%     U = a;
% else
%     U= uint8(zeros(41,1));
% end
end

== matlab function SIMQGC/UDPReadFromQGC/Subsystem/data_transfer ==
  data: data input; index output; control output
function [index,control] = fcn(data)
if data(1,1) ~= 68 || data(2,1) ~= 65
    index = 999;
    control = single([-999;-999;-999;-999;-999;-999;-999;-999]);
    return
end
index = double(data(6));
control = typecast(data(10 : 41,1),'single');
end
